simulink model "zad7"  (R2022b)
settings: Solver=VariableStepAuto  StartTime=0.0  StopTime=100  RelTol=1e-3
values from neighbouring files (symbols this model uses):
  a0 = 0.000641026    [parameters.m]
  a1 = 0.0224359    [parameters.m]
  a2 = 0.260256    [parameters.m]
  Tp = 1    [parameters.m]
settings Model: Creator=Mat  LastModifiedBy=Mat

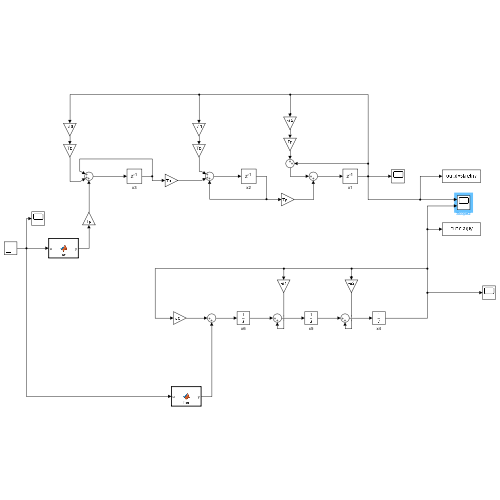
[thumbnail: Simulink's stored preview of the top-level diagram]
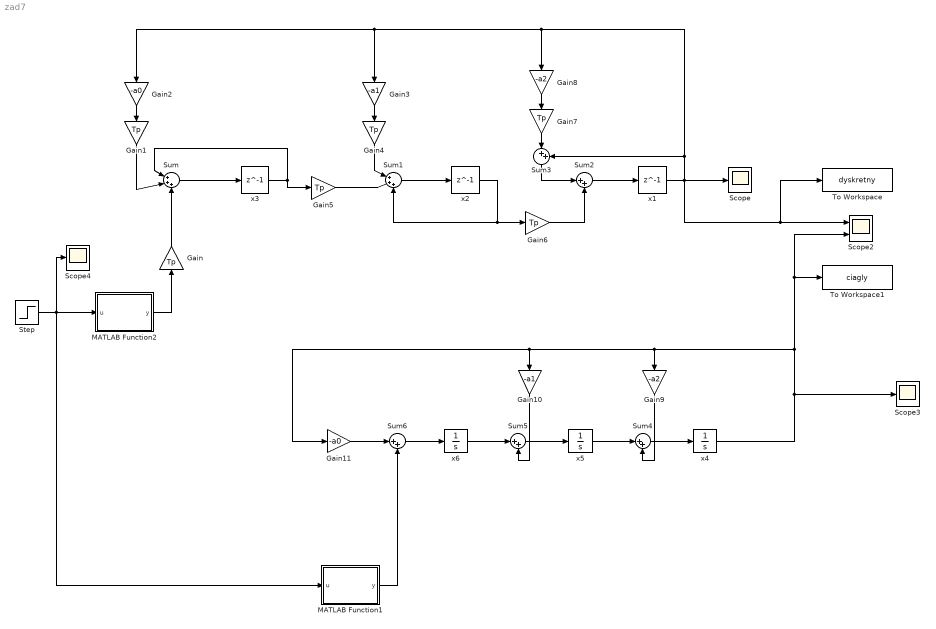
== system zad7 ==
  Gain{,1,4..7} (6 alike) : Gain  Gain=Tp
  Gain10 : Gain  Gain=-a1
  Gain11 : Gain  Gain=-a0
  Gain2 : Gain  Gain=-a0
  Gain3 : Gain  Gain=-a1
  Gain8 : Gain  Gain=-a2
  Gain9 : Gain  Gain=-a2
  MATLAB Function1 : MATLAB Function  TreatAsAtomicUnit=on
  MATLAB Function2 : MATLAB Function  TreatAsAtomicUnit=on
  Scope : Scope
  Scope2 : Scope  NumInputPorts=2
  Scope3 : Scope
  Scope4 : Scope
  Step : Step  Time=0  SampleTime=Tp
  Sum : Sum  Inputs=|+++
  Sum1 : Sum  Inputs=|+++
  Sum{2..6} (5 alike) : Sum  Inputs=|++
  To Workspace : ToWorkspace  VariableName=dyskretny  SaveFormat=Timeseries  SampleTime=-1
  To Workspace1 : ToWorkspace  VariableName=ciagly  SaveFormat=Timeseries  SampleTime=-1
  x1 : Delay  DelayLength=1  InitialCondition=0  SampleTime=Tp
  x2 : Delay  DelayLength=1  InitialCondition=0  SampleTime=Tp
  x3 : Delay  DelayLength=1  InitialCondition=0  SampleTime=Tp
  x4 : Integrator
  x5 : Integrator
  x6 : Integrator
  wires:
  MATLAB Function2/1(y) -> Gain/1
  x3/1 -> Gain5/1, Sum/1
  Gain/1 -> Sum/3
  x1/1 -> To Workspace/1, Scope2/1, Scope/1, Gain8/1, Gain3/1, Gain2/1, Sum3/2
  Gain2/1 -> Gain1/1
  Gain1/1 -> Sum/2
  Sum/1 -> x3/1
  Gain3/1 -> Gain4/1
  Gain4/1 -> Sum1/1
  x2/1 -> Gain6/1, Sum1/3
  Gain5/1 -> Sum1/2
  Sum1/1 -> x2/1
  Gain6/1 -> Sum2/2
  Sum2/1 -> x1/1
  Sum3/1 -> Sum2/1
  Gain8/1 -> Gain7/1
  Gain7/1 -> Sum3/1
  Sum6/1 -> x6/1
  x4/1 -> Scope3/1, To Workspace1/1, Scope2/2, Gain10/1, Gain11/1, Gain9/1
  Sum4/1 -> x4/1
  x5/1 -> Sum4/1
  x6/1 -> Sum5/1
  Step/1 -> MATLAB Function1/1(u), Scope4/1, MATLAB Function2/1(u)
  Gain10/1 -> Sum5/2
  MATLAB Function1/1(y) -> Sum6/2
  Gain9/1 -> Sum4/2
  Sum5/1 -> x5/1
  Gain11/1 -> Sum6/1

== matlab function zad7/MATLAB Function2 ==
  data: u input; y output
function y = fcn(u)
b0 = 0.000897436;
alfa1 = 1.3;
alfa2 = 1.1;
alfa3 = -1.15;
alfa4 = -0.9;
y = b0*(alfa1*u+alfa2*u^2+alfa3*u^3+alfa4*u^4);
end

== matlab function zad7/MATLAB Function1 ==
  data: u input; y output
function y = fcn(u)
b0 = 0.000897436;
alfa1 = 1.3;
alfa2 = 1.1;
alfa3 = -1.15;
alfa4 = -0.9;
y = b0*(alfa1*u+alfa2*u^2+alfa3*u^3+alfa4*u^4);
end
